simulink model "smtest"  (Simulink 8.3)
settings: Solver=ode45  StartTime=0.0  StopTime=10.0  RelTol=1e-3
settings Model: Creator=baidx  LastModifiedBy=baidx
settings DataIOCC: SignalLoggingSaveFormat=Dataset
settings DebuggingCC: UnderspecifiedInitializationDetection=Simplified  StateNameClashWarn=none
settings GRTTargetCC: CombineOutputUpdateFcns=on  GRTInterface=off

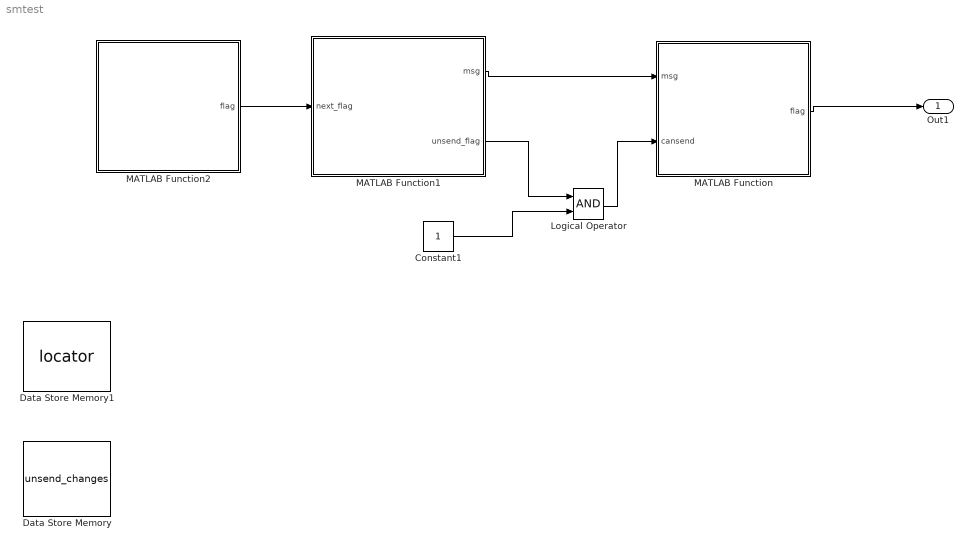
== system smtest ==
  Constant1 : Constant  OutDataTypeStr=boolean
  Data Store Memory : DataStoreMemory  DataStoreName=unsend_changes  ReadBeforeWriteMsg=warning  WriteAfterWriteMsg=warning  WriteAfterReadMsg=warning  InitialValue=10  OutDataTypeStr=double
  Data Store Memory1 : DataStoreMemory  DataStoreName=locator  ReadBeforeWriteMsg=warning  WriteAfterWriteMsg=warning  WriteAfterReadMsg=warning  OutDataTypeStr=double
  Logical Operator : Logic  AllPortsSameDT=off  OutDataTypeStr=boolean
  MATLAB Function : MATLAB Function  TreatAsAtomicUnit=on
  MATLAB Function1 : MATLAB Function  TreatAsAtomicUnit=on
  MATLAB Function2 : MATLAB Function  TreatAsAtomicUnit=on
  Out1 : Outport
  wires:
  Logical Operator/1 -> MATLAB Function/2(cansend)
  MATLAB Function/1(flag) -> Out1/1
  MATLAB Function1/1(msg) -> MATLAB Function/1(msg)
  MATLAB Function1/2(unsend_flag) -> Logical Operator/1
  Constant1/1 -> Logical Operator/2
  MATLAB Function2/1(flag) -> MATLAB Function1/1(next_flag)

== matlab function MATLAB Function1 ==
  data: next_flag input double; msg output double; unsend_flag output double; unsend_changes data_store_memory double

function [msg,unsend_flag] = fcn2(next_flag)
   global unsend_changes;
   if unsend_changes>0 && next_flag==true
       msg=unsend_changes;
       unsend_changes=unsend_changes-1;
       unsend_flag=true;
 
   else
       msg=0;
       unsend_flag=false;
   end
end
   
   
   
   
%#codegen

== matlab function MATLAB Function ==
  data: msg input double size=1; cansend input boolean size=1; flag output double; locator data_store_memory double
function flag = sfunt(msg,cansend) %定义函数名称：sfuntenden
    global locator;
    if cansend==1
        locator=locator+msg;
        flag=1;
    else
        flag=0;
    end

end

== matlab function MATLAB Function2 ==
  data: flag output double; locator data_store_memory double; unsend_changes data_store_memory double
function flag=init
%#codegen
global locator
global unsend_changes
locator=0;
unsend_changes=10;
flag=1;
end
